simulink model "modelRamieniaTest"  (R2015a)
settings: Solver=ode45  StartTime=0.0  StopTime=200  FixedStep=0.1  RelTol=1e-3
values from neighbouring files (symbols this model uses):
  I1 = 1.8273e-08    [ParametryDoSymulacji.m]
  I2 = 0.0048    [ParametryDoSymulacji.m]
  J1 = Jr + mw * r*r    (= 0.541666666667)    [LP1.m]    (also in ParametryDoSymulacji.m = 0.416666666667; USImodel.m = 0.416666666667; wskaJak1.m = 0.416666666667; wskaJak2.m = 0.416666666667)
  J2 = Jr + mw * r*r    (= 0.541666666667)    [ParametryDoSymulacji.m]    (also in USImodel.m; wskaJak1.m; wskaJak2.m; wskaJak3.m)
  k = 0.1    [LP1.m]    (also in ParametryDoSymulacji.m; USImodel.m; wskaJak1.m; wskaJak2.m)
  ke = 5    [LP1.m]    (also in ParametryDoSymulacji.m; USImodel.m; wskaJak1.m; wskaJak2.m)
  L = 0.1    [LP1.m]    (also in ParametryDoSymulacji.m; USImodel.m; wskaJak1.m; wskaJak2.m)
  P1 = 0.9525    [ParametryDoSymulacji.m]
  P2 = 0.7384    [ParametryDoSymulacji.m]
  R = 2    [LP1.m]    (also in ParametryDoSymulacji.m; USImodel.m; wskaJak1.m; wskaJak2.m)
libraries: simulink x10, simulink_extras x1
settings Model: Creator=Kamil  LastModifiedBy=konra

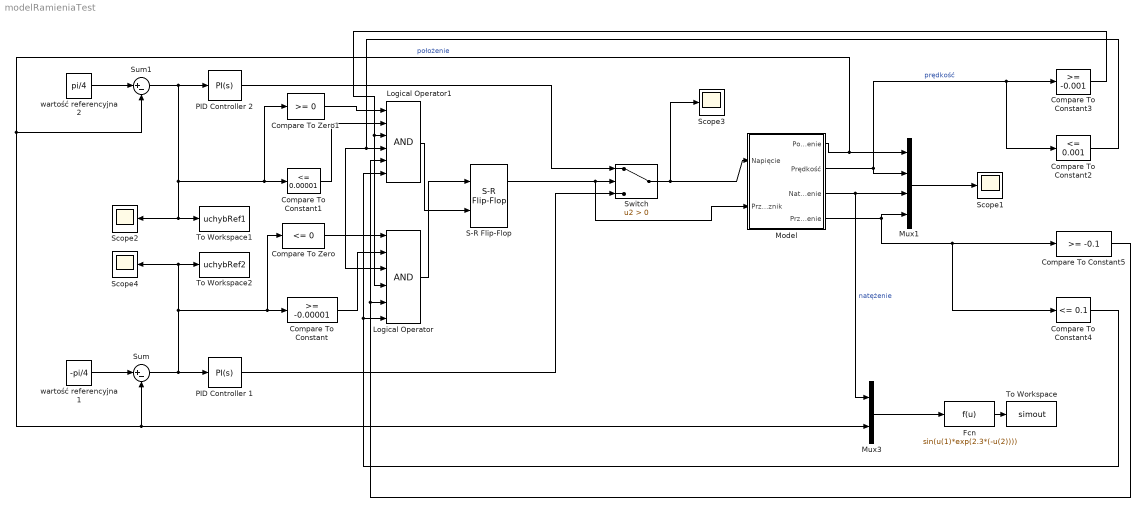
== system modelRamieniaTest ==
  Compare To Constant : simulink/Logic and Bit Operations/Compare To Constant  relop=>=  const=-0.00001  OutDataTypeStr=boolean
  Compare To Constant1 : simulink/Logic and Bit Operations/Compare To Constant  relop=<=  const=0.00001  OutDataTypeStr=boolean
  Compare To Constant2 : simulink/Logic and Bit Operations/Compare To Constant  relop=<=  const=0.001  OutDataTypeStr=boolean
  Compare To Constant3 : simulink/Logic and Bit Operations/Compare To Constant  relop=>=  const=-0.001  OutDataTypeStr=boolean
  Compare To Constant4 : simulink/Logic and Bit Operations/Compare To Constant  relop=<=  const=0.1  OutDataTypeStr=boolean
  Compare To Constant5 : simulink/Logic and Bit Operations/Compare To Constant  relop=>=  const=-0.1  OutDataTypeStr=boolean
  Compare To Zero : simulink/Logic and Bit Operations/Compare To Zero  relop=<=  OutDataTypeStr=boolean
  Compare To Zero1 : simulink/Logic and Bit Operations/Compare To Zero  relop=>=  OutDataTypeStr=boolean
  Fcn : Fcn  Expr=sin(u(1)*exp(2.3*(-u(2))))
  Logical Operator : Logic  Inputs=6  AllPortsSameDT=off  OutDataTypeStr=boolean
  Logical Operator1 : Logic  Inputs=6  AllPortsSameDT=off  OutDataTypeStr=boolean
  Model : Subsystem
  Mux1 : Mux
  Mux3 : Mux  Inputs=2
  PID Controller 1 : simulink/Continuous/PID Controller  Controller=PI  TimeDomain=Continuous-time  SampleTime=-1  IntegratorMethod=Forward Euler  FilterMethod=Forward Euler  Form=Parallel  UseFilter=on  ControllerParametersSource=internal  P=P2  I=I2  D=0  N=100  InitialConditionSource=internal  InitialConditionForIntegrator=0  InitialConditionForFilter=0  ExternalReset=none  LimitOutput=off  UpperSaturationLimit=inf  LowerSaturationLimit=-inf  LinearizeAsGain=on  AntiWindupMode=none  Kb=1  TrackingMode=off  Kt=1  PParamMin=[]  PParamMax=[]  IParamMin=[]  IParamMax=[]  DParamMin=[]  DParamMax=[]  NParamMin=[]  NParamMax=[]  KbParamMin=[]  KbParamMax=[]  KtParamMin=[]  KtParamMax=[]  POutMin=[]  POutMax=[]  IOutMin=[]  IOutMax=[]  DOutMin=[]  DOutMax=[]  NOutMin=[]  NOutMax=[]  KbOutMin=[]  KbOutMax=[]  KtOutMin=[]  KtOutMax=[]  IntegratorOutMin=[]  IntegratorOutMax=[]  FilterOutMin=[]  FilterOutMax=[]  SumOutMin=[]  SumOutMax=[]  SumI1OutMin=[]  SumI1OutMax=[]  SumI2OutMin=[]  SumI2OutMax=[]  SumI3OutMin=[]  SumI3OutMax=[]  SumDOutMin=[]  SumDOutMax=[]  SaturationOutMin=[]  SaturationOutMax=[]  IntegratorContinuousStateAttributes=''  IntegratorStateMustResolveToSignalObject=off  IntegratorRTWStateStorageClass=Auto  FilterContinuousStateAttributes=''  FilterStateMustResolveToSignalObject=off  FilterRTWStateStorageClass=Auto  DifferentiatorICPrevScaledInput=0  DifferentiatorOutMin=[]  DifferentiatorOutMax=[]
  PID Controller 2 : simulink/Continuous/PID Controller  Controller=PI  TimeDomain=Continuous-time  SampleTime=-1  IntegratorMethod=Forward Euler  FilterMethod=Forward Euler  Form=Parallel  UseFilter=on  ControllerParametersSource=internal  P=P1  I=I1  D=0.650317519793469  N=3.71494151618387  InitialConditionSource=internal  InitialConditionForIntegrator=0  InitialConditionForFilter=0  ExternalReset=none  LimitOutput=off  UpperSaturationLimit=inf  LowerSaturationLimit=-inf  LinearizeAsGain=on  AntiWindupMode=none  Kb=1  TrackingMode=off  Kt=1  PParamMin=[]  PParamMax=[]  IParamMin=[]  IParamMax=[]  DParamMin=[]  DParamMax=[]  NParamMin=[]  NParamMax=[]  KbParamMin=[]  KbParamMax=[]  KtParamMin=[]  KtParamMax=[]  POutMin=[]  POutMax=[]  IOutMin=[]  IOutMax=[]  DOutMin=[]  DOutMax=[]  NOutMin=[]  NOutMax=[]  KbOutMin=[]  KbOutMax=[]  KtOutMin=[]  KtOutMax=[]  IntegratorOutMin=[]  IntegratorOutMax=[]  FilterOutMin=[]  FilterOutMax=[]  SumOutMin=[]  SumOutMax=[]  SumI1OutMin=[]  SumI1OutMax=[]  SumI2OutMin=[]  SumI2OutMax=[]  SumI3OutMin=[]  SumI3OutMax=[]  SumDOutMin=[]  SumDOutMax=[]  SaturationOutMin=[]  SaturationOutMax=[]  IntegratorContinuousStateAttributes=''  IntegratorStateMustResolveToSignalObject=off  IntegratorRTWStateStorageClass=Auto  FilterContinuousStateAttributes=''  FilterStateMustResolveToSignalObject=off  FilterRTWStateStorageClass=Auto  DifferentiatorICPrevScaledInput=0  DifferentiatorOutMin=[]  DifferentiatorOutMax=[]
  S-R Flip-Flop : simulink_extras/Flip Flops/S-R Flip-Flop  initial_condition=0
  Scope{1..4} (4 alike) : Scope
      Scope1 settings: ShowLegends=on  MaxDataPoints=10000
      Scope3 settings: SaveName=ScopeData3
      Scope4 settings: SaveName=ScopeData2
  Sum : Sum  Inputs=|+-
  Sum1 : Sum  Inputs=|+-
  Switch : Switch  Criteria=u2 > Threshold
  To Workspace : ToWorkspace  VariableName=simout  SaveFormat=Timeseries  SampleTime=-1
  To Workspace1 : ToWorkspace  VariableName=uchybRef1  SaveFormat=Timeseries  SampleTime=-1
  To Workspace2 : ToWorkspace  VariableName=uchybRef2  SaveFormat=Timeseries  SampleTime=-1
  wartość referencyjna 1 : Constant  Value=-pi/4
  wartość referencyjna 2 : Constant  Value=pi/4
  wires:
  wartość referencyjna 1/1 -> Sum/1
  Sum/1 -> Compare To Zero/1, Compare To Constant/1, Scope4/1, To Workspace2/1, PID Controller 1/1
  Fcn/1 -> To Workspace/1
  Mux3/1 -> Fcn/1
  wartość referencyjna 2/1 -> Sum1/1
  Sum1/1 -> To Workspace1/1, Scope2/1, Compare To Constant1/1, Compare To Zero1/1, PID Controller 2/1
  PID Controller 1/1 -> Switch/3
  PID Controller 2/1 -> Switch/1
  S-R Flip-Flop/1 -> Model/2(Przelacznik), Switch/2
  Switch/1 -> Model/1(Napięcie), Scope3/1
  Compare To Constant/1 -> Logical Operator/2
  Compare To Zero/1 -> Logical Operator/1
  Logical Operator/1 -> S-R Flip-Flop/1
  Compare To Zero1/1 -> Logical Operator1/1
  Compare To Constant1/1 -> Logical Operator1/2
  Logical Operator1/1 -> S-R Flip-Flop/2
  Model/1(Położenie) -> Mux3/2, Sum/2, Sum1/2, Mux1/1  "położenie"
  Model/3("Natężenie ") -> Mux1/3, Mux3/1  "natężenie"
  Model/2(Prędkość) -> Mux1/2, Compare To Constant2/1, Compare To Constant3/1  "prędkość"
  Mux1/1 -> Scope1/1
  Compare To Constant3/1 -> Logical Operator/4, Logical Operator1/3
  Compare To Constant2/1 -> Logical Operator1/4, Logical Operator/3
  Compare To Constant5/1 -> Logical Operator/5, Logical Operator1/5
  Compare To Constant4/1 -> Logical Operator/6, Logical Operator1/6
  Model/4(Przyspieszenie) -> Compare To Constant4/1, Compare To Constant5/1, Mux1/4

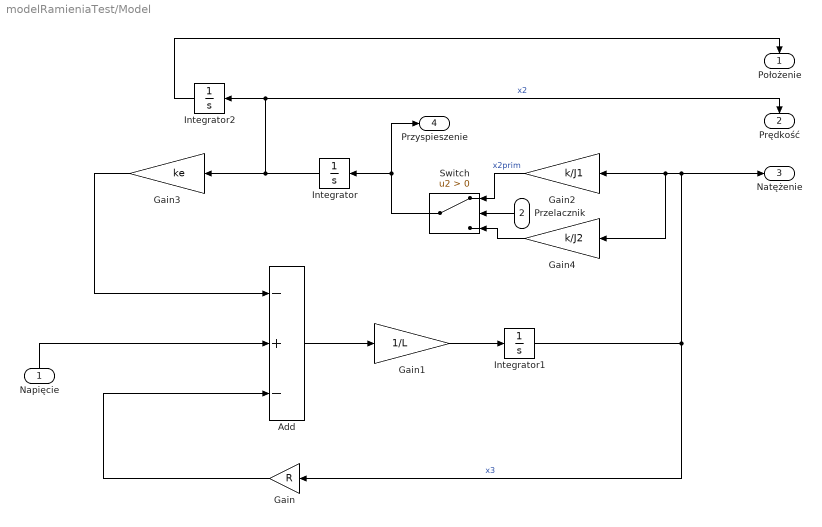
== system modelRamieniaTest/Model ==
  Napięcie : Inport
  Przelacznik : Inport  Port=2
  Add : Sum  Inputs=-+-
  Gain : Gain  Gain=R
  Gain1 : Gain  Gain=1/L
  Gain2 : Gain  Gain=k/J1
  Gain3 : Gain  Gain=ke
  Gain4 : Gain  Gain=k/J2
  Integrator : Integrator
  Integrator1 : Integrator
  Integrator2 : Integrator  InitialCondition=-pi/4
  Switch : Switch  Criteria=u2 > Threshold
  Położenie : Outport
  Prędkość : Outport  Port=2
  "Natężenie " : Outport  Port=3
  Przyspieszenie : Outport  Port=4
  wires:
  Add/1 -> Gain1/1
  Gain1/1 -> Integrator1/1
  Gain3/1 -> Add/1
  Integrator/1 -> Prędkość/1, Integrator2/1, Gain3/1  "x2"
  Integrator2/1 -> Położenie/1
  Gain/1 -> Add/3
  Integrator1/1 -> "Natężenie "/1, Gain4/1, Gain2/1, Gain/1  "x3"
  Napięcie/1 -> Add/2
  Przelacznik/1 -> Switch/2
  Gain4/1 -> Switch/3
  Gain2/1 -> Switch/1  "x2prim"
  Switch/1 -> Przyspieszenie/1, Integrator/1
